simulink library "ODEHubs_components"  (R2020b)
settings: Solver=VariableStepAuto  StartTime=0.0  StopTime=10.0  RelTol=1e-3
values from neighbouring files (symbols this model uses):
  I = aux    [EH_definition_Simulink.m]
  O = aux    [EH_definition_Simulink.m]
undefined symbols (not defined in the file or in its folder): AbsorptionChiller, beta1, BiomassBoiler, Boiler, CN0, CombinedHeatAndPower, cpa, DesalinationPlant, dispatch_factor, DN0, efficiency, HeatPump, IrrigationPump, Low, Low1, Low2, Max_in, Max_out, Min_in, NanofiltrationPlant, PVModules, r_c, r_d, ReversibleHeatPump, SolarCollector, StorageSystem, T_muestreo, Tm, Up, Up1, Up2
(part 1 of 2)
settings Model: Creator=Usuario  LastModifiedBy=Javi
settings SFSimCC: CustomCodeUndefinedFunction=UseInterfaceOnly

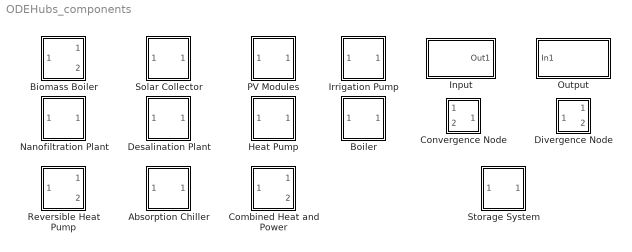
== system ODEHubs_components ==
  Absorption Chiller : Subsystem  mask{label=AbsorptionChiller, n=0, nI=1:1, tI="H", nO=1:1, tO="C", sO=1, Dimin=0, Dimax=0, Domin=0, Domax=0, nd=0}
      mask prompts: label "ID label:"; n "Number:"; Dimin "Input flow(s) lower bound (Dimin):"; Dimax "Input flow(s) upper bound (Dimax):"; Domin "Output flow(s) lower bounds (Domin):"; Domax "Output flow(s) upper bounds (Domax):"; nd "Conversion factor(s):"
      mask init:
      | %% Update user defined data from library
      | parent=libinfo(gcb);
      | if ~isempty(parent)
      | s_new=get_param(parent.ReferenceBlock,'UserData');
      | s_old=get_param(gcb,'UserData');
      | 
      | % Remove overlapping fields from first struct
      | s_merged = rmfield(s_old, intersect(fieldnames(s_old), fieldnames(s_new)));
      | 
      | % Obtain all unique names of remaining fields
      | names = [fieldnames(s_merged); fieldnames(s_new)];
      | 
      | % Merge both structs
      | s_merged = cell2struct([struct2cell(s_merged); struct2cell(s_new)], names, 1);
      | 
      | set_param(gcb,'UserData',s_merged);
      | set_param(gcb, 'UserDataPersistent', 'on');
      | end
      mask DialogControl DescGroupVar Prompt: Description
      mask DialogControl DescTextVar Prompt: Device description
      mask DialogControl Container3 Prompt: Device
      mask DialogControl ParameterGroupVar Prompt: Model
      mask Display:
      | %%Draw icon
      | ud = get_param(gcb,'UserData');
      | image(ud.icon);
      | 
      | 
      | %%Update label
      | subsys=find_system(gcs,...
      |     'LookUnderMasks','on',...
      |     'FollowLinks','on','BlockType','SubSystem');
      | UD=get_param(subsys,'UserData');
      | devs={};
      | for i=1:length(UD)
      |     if isfield(UD{i},'type')
      |         if UD{i}.type=='D'
      |             devs{end+1}=subsys{i}; %filter devices (D)
      |         end
      |     end
      | end
      | 
      | names=get_param(devs,'Name'); %all dev names
      | names=names(~cellfun(@isempty,erase(names,get_param(gcb,'Name')))); %remove this block
      | labels=matlab.lang.makeValidName(names); %all, but this block, dev labels
      | set_param(gcb,'label',matlab.lang.makeUniqueStrings(... %ensure uniqueness
      |                       matlab.lang.makeValidName(get_param(gcb,'Name')),...
      |                                                 labels))
  Biomass Boiler : Subsystem  mask{label=BiomassBoiler, n=0, nI=1:1, tI="B", nO=1:2, tO=["H";"G"], sO=[1 1], Dimin=0, Dimax=0, Domin=0, Domax=0, nd=0}
      mask prompts: label "ID label:"; n "Number:"; Dimin "Input flow(s) lower bound (Dimin):"; Dimax "Input flow(s) upper bound (Dimax):"; Domin "Output flow(s) lower bounds (Domin):"; Domax "Output flow(s) upper bounds (Domax):"; nd "Conversion factor(s):"
      mask init: same as ODEHubs_components/Absorption Chiller
      mask DialogControl DescGroupVar Prompt: Description
      mask DialogControl DescTextVar Prompt: Device description
      mask DialogControl Container3 Prompt: Device
      mask DialogControl ParameterGroupVar Prompt: Model
      mask Display:
      | %%Draw icon
      | ud = get_param(gcb,'UserData');
      | image(ud.icon);
      | 
      | 
      | %%Update label
      | subsys=find_system(gcs,...
      |     'LookUnderMasks','on',...
      |     'FollowLinks','on','BlockType','SubSystem');
      | UD=get_param(subsys,'UserData');
      | devs={};
      | for i=1:length(UD)
      |     if isfield(UD{i},'type')
      |         if UD{i}.type=='D'
      |             devs{end+1}=subsys{i}; %filter devices (D)
      |         end
      |     end
      | end
      | 
      | names=get_param(devs,'Name'); %all dev names
      | names=names(~cellfun(@isempty,erase(names,get_param(gcb,'Name')))); %remove this block
      | labels=matlab.lang.makeValidName(names); %all, but this block, dev labels
      | set_param(gcb,'label',matlab.lang.makeUniqueStrings(... %ensure uniqueness
      |                       matlab.lang.makeValidName(get_param(gcb,'Name')),...
      |                                                 labels))
  Boiler : Subsystem  mask{label=Boiler, n=0, nI=1:1, tI="P", nO=1:1, tO="H", sO=1, Dimin=0, Dimax=0, Domin=0, Domax=0, nd=0}
      mask prompts: label "ID label:"; n "Number:"; Dimin "Input flow(s) lower bound (Dimin):"; Dimax "Input flow(s) upper bound (Dimax):"; Domin "Output flow(s) lower bounds (Domin):"; Domax "Output flow(s) upper bounds (Domax):"; nd "Conversion factor(s):"
      mask init: same as ODEHubs_components/Absorption Chiller
      mask DialogControl DescGroupVar Prompt: Description
      mask DialogControl DescTextVar Prompt: Device description
      mask DialogControl Container3 Prompt: Device
      mask DialogControl ParameterGroupVar Prompt: Model
      mask Display:
      | %%Draw icon
      | ud = get_param(gcb,'UserData');
      | image(ud.icon);
      | 
      | 
      | %%Update label
      | subsys=find_system(gcs,...
      |     'LookUnderMasks','on',...
      |     'FollowLinks','on','BlockType','SubSystem');
      | UD=get_param(subsys,'UserData');
      | devs={};
      | for i=1:length(UD)
      |     if isfield(UD{i},'type')
      |         if UD{i}.type=='D'
      |             devs{end+1}=subsys{i}; %filter devices (D)
      |         end
      |     end
      | end
      | 
      | names=get_param(devs,'Name'); %all dev names
      | names=names(~cellfun(@isempty,erase(names,get_param(gcb,'Name')))); %remove this block
      | labels=matlab.lang.makeValidName(names); %all, but this block, dev labels
      | set_param(gcb,'label',matlab.lang.makeUniqueStrings(... %ensure uniqueness
      |                       matlab.lang.makeValidName(get_param(gcb,'Name')),...
      |                                                 labels))
  Combined Heat and Power : Subsystem  mask{label=CombinedHeatAndPower, n=0, nI=1:1, tI="P", nO=1:2, tO=["H";"E"], sO=[1 1], Dimin=0, Dimax=0, Domin=0, Domax=0, nd=0}
      mask prompts: label "ID label:"; n "Number:"; Dimin "Input flow(s) lower bound (Dimin):"; Dimax "Input flow(s) upper bound (Dimax):"; Domin "Output flow(s) lower bounds (Domin):"; Domax "Output flow(s) upper bounds (Domax):"; nd "Conversion factor(s):"
      mask init: same as ODEHubs_components/Absorption Chiller
      mask DialogControl DescGroupVar Prompt: Description
      mask DialogControl DescTextVar Prompt: Device description
      mask DialogControl Container3 Prompt: Device
      mask DialogControl ParameterGroupVar Prompt: Model
      mask Display:
      | %%Draw icon
      | ud = get_param(gcb,'UserData');
      | image(ud.icon);
      | 
      | 
      | %%Update label
      | subsys=find_system(gcs,...
      |     'LookUnderMasks','on',...
      |     'FollowLinks','on','BlockType','SubSystem');
      | UD=get_param(subsys,'UserData');
      | devs={};
      | for i=1:length(UD)
      |     if isfield(UD{i},'type')
      |         if UD{i}.type=='D'
      |             devs{end+1}=subsys{i}; %filter devices (D)
      |         end
      |     end
      | end
      | 
      | names=get_param(devs,'Name'); %all dev names
      | names=names(~cellfun(@isempty,erase(names,get_param(gcb,'Name')))); %remove this block
      | labels=matlab.lang.makeValidName(names); %all, but this block, dev labels
      | set_param(gcb,'label',matlab.lang.makeUniqueStrings(... %ensure uniqueness
      |                       matlab.lang.makeValidName(get_param(gcb,'Name')),...
      |                                                 labels))
  Convergence Node : Subsystem  mask{ID=CN0, n=0, Inputs=2}
      mask prompts: ID "ID label:"; n "Number:"; Inputs "Number of input flows:"
      mask init:
      | %% Update user defined data from library
      | parent=libinfo(gcb);
      | if ~isempty(parent)
      | s_new=get_param(parent.ReferenceBlock,'UserData');
      | s_old=get_param(gcb,'UserData');
      | 
      | % Remove overlapping fields from first struct
      | s_merged = rmfield(s_old, intersect(fieldnames(s_old), fieldnames(s_new)));
      | 
      | % Obtain all unique names of remaining fields
      | names = [fieldnames(s_merged); fieldnames(s_new)];
      | 
      | % Merge both structs
      | s_merged = cell2struct([struct2cell(s_merged); struct2cell(s_new)], names, 1);
      | 
      | set_param(gcb,'UserData',s_merged);
      | set_param(gcb, 'UserDataPersistent', 'on');
      | end
      | 
      | %%Update label
      | n = get_param(gcb,'n');
      | set_param(gcb,'ID',strcat('CN',num2str(n)));
      | 
      | %Update subsystem structure
      | blocks=find_system(gcb,...
      |         'LookUnderMasks','on',...
      |         'FollowLinks','on','BlockType','Inport');
      | lines=find_system(gcb,...
      |         'LookUnderMasks','on',...
      |         'FollowLinks','on','FindAll','On','type','line'); 
      | 
      | if Inputs~=length(blocks)
      |     
      |     %Delete all input ports
      |     delete_block(blocks)
      |     
      |     %Delete all the lines
      |     delete_line(lines)
      |     
      |     %Set sum block inputs
      |     set_param(strcat(gcb,'/Sum'),'Inputs',num2str(Inputs))
      |     
      |     %Build new inputs and lines
      |     for k=1:Inputs
      |         newblock=[gcb,char(strcat('/In',num2str(k)))];
      |         add_block('built-in/Inport',newblock);
      |         P0=get_param(newblock,'position');
      |         P=P0;
      |         P(1)=P0(1)+8; %left
      |         P(2)=P0(2)+18+k*20-100; %top
      |         P(3)=P0(3)-8; %right
      |         P(4)=P0(4)-18+k*20-100; %bottom
      |         set_param(newblock,'position',P);
      |         add_line(gcb,...
      |             strcat('In',num2str(k),'/1'),... %out
      |             strcat('Sum/',num2str(k)),...%in
      |             'autorouting','on')
      |     end
      |     add_line(gcb,...
      |         'Sum/1',... %out
      |         'Out1/1',...%in
      |         'autorouting','on')
      | end
      mask DialogControl DescGroupVar Prompt: Description
      mask DialogControl DescTextVar Prompt: Convergence node whose output is the sum of all the input flows
      mask Display:
      | icon=sprintf('\\fontname{Palatino Linotype}CN %s',n);
      | disp(icon, 'texmode','on');
      | plot(sin(0:0.0001:2*pi),cos(0:0.0001:2*pi))
  Desalination Plant : Subsystem  mask{label=DesalinationPlant, n=0, nI=1:1, tI="S", nO=1:1, tO="W", sO=1, Dimin=0, Dimax=0, Domin=0, Domax=0, nd=0}
      mask prompts: label "ID label:"; n "Number:"; Dimin "Input flow(s) lower bound (Dimin):"; Dimax "Input flow(s) upper bound (Dimax):"; Domin "Output flow(s) lower bounds (Domin):"; Domax "Output flow(s) upper bounds (Domax):"; nd "Conversion factor(s):"
      mask init: same as ODEHubs_components/Absorption Chiller
      mask DialogControl DescGroupVar Prompt: Description
      mask DialogControl DescTextVar Prompt: Device description
      mask DialogControl Container3 Prompt: Device
      mask DialogControl ParameterGroupVar Prompt: Model
      mask Display:
      | %%Draw icon
      | ud = get_param(gcb,'UserData');
      | image(ud.icon);
      | 
      | 
      | %%Update label
      | subsys=find_system(gcs,...
      |     'LookUnderMasks','on',...
      |     'FollowLinks','on','BlockType','SubSystem');
      | UD=get_param(subsys,'UserData');
      | devs={};
      | for i=1:length(UD)
      |     if isfield(UD{i},'type')
      |         if UD{i}.type=='D'
      |             devs{end+1}=subsys{i}; %filter devices (D)
      |         end
      |     end
      | end
      | 
      | names=get_param(devs,'Name'); %all dev names
      | names=names(~cellfun(@isempty,erase(names,get_param(gcb,'Name')))); %remove this block
      | labels=matlab.lang.makeValidName(names); %all, but this block, dev labels
      | set_param(gcb,'label',matlab.lang.makeUniqueStrings(... %ensure uniqueness
      |                       matlab.lang.makeValidName(get_param(gcb,'Name')),...
      |                                                 labels))
  Divergence Node : Subsystem  mask{ID=DN0, n=0, Outputs=2}
      mask prompts: ID "ID label:"; n "Number:"; Outputs "Number of output flows:"
      mask init:
      | %% Update user defined data from library
      | parent=libinfo(gcb);
      | if ~isempty(parent)
      | s_new=get_param(parent.ReferenceBlock,'UserData');
      | s_old=get_param(gcb,'UserData');
      | 
      | % Remove overlapping fields from first struct
      | s_merged = rmfield(s_old, intersect(fieldnames(s_old), fieldnames(s_new)));
      | 
      | % Obtain all unique names of remaining fields
      | names = [fieldnames(s_merged); fieldnames(s_new)];
      | 
      | % Merge both structs
      | s_merged = cell2struct([struct2cell(s_merged); struct2cell(s_new)], names, 1);
      | 
      | set_param(gcb,'UserData',s_merged);
      | set_param(gcb, 'UserDataPersistent', 'on');
      | end
      | 
      | %%Update label
      | n = get_param(gcb,'n');
      | set_param(gcb,'ID',strcat('DN',num2str(n)));
      | 
      | %%Update subsys structure
      | blocks1=find_system(gcb,...
      |         'LookUnderMasks','on',...
      |         'FollowLinks','on','BlockType','Gain');
      | blocks2=find_system(gcb,...
      |         'LookUnderMasks','on',...
      |         'FollowLinks','on','BlockType','Outport');
      | lines=find_system(gcb,...
      |         'LookUnderMasks','on',...
      |         'FollowLinks','on','FindAll','On','type','line'); 
      | 
      | if Outputs~=length(blocks2)
      |     
      |     %Delete all gain ports
      |     delete_block(blocks1)
      |     
      |     %Delete all output ports
      |     delete_block(blocks2)
      |     
      |     %Delete all the lines
      |     delete_line(lines)
      |     
      |     %Set mux and demux ports
      |     set_param(strcat(gcb,'/Mux'),'Inputs',num2str(Outputs))
      |     set_param(strcat(gcb,'/Demux'),'Outputs',num2str(Outputs))
      |     
      |     %Build new inputs and lines
      |     for k=1:Outputs
      |         
      |         %Add output ports
      |         newblock=[gcb,char(strcat('/Out',num2str(k)))];
      |         add_block('built-in/Outport',newblock);
      |         P0=get_param(newblock,'position');
      |         P=P0;
      |         P(1)=P0(1)+8; %left
      |         P(2)=P0(2)+18-80+k*20; %top
      |         P(3)=P0(3)-8; %right
      |         P(4)=P0(4)-18-80+k*20; %bottom
      |         set_param(newblock,'position',P);
      |         
      |         %Add gains
      |         newblock=[gcb,char(strcat('/Gain',num2str(k)))];
      |         add_block('built-in/Gain',newblock);
      |         P0=get_param(newblock,'position');
      |         P=P0;
      |         P(1)=P0(1)+8-40; %left
      |         P(2)=P0(2)+18-80+k*20; %top
      |         P(3)=P0(3)-8-40; %right
      |         P(4)=P0(4)-18-80+k*20; %bottom
      |         set_param(newblock,'position',P);
      |         %set equal default gains
      |         set_param(strcat(gcb,'/Gain',num2str(k)),'Gain',num2str(1/Outputs))
      |         
      |         %link in to mux ports
      |         add_line(gcb,...
      |             'In1/1',... %out
      |             strcat('Mux/',num2str(k)),...%in
      |             'autorouting','on')
      |         %link demux ports to gains
      |         add_line(gcb,...
      |             strcat('Demux/',num2str(k)),... %out
      |             strcat('Gain',num2str(k),'/1'),...%in
      |             'autorouting','on')
      |         %link gains to output ports
      |         add_line(gcb,...
      |             strcat('Gain',num2str(k),'/1'),... %out
      |             strcat('Out',num2str(k),'/1'),...%in
      |             'autorouting','on')
      |     end
      |     %link mux to demux
      |     add_line(gcb,...
      |         'Mux/1',... %in
      |         'Demux/1',...%out
      |         'autorouting','on')
      | end
      mask DialogControl DescGroupVar Prompt: Description
      mask DialogControl DescTextVar Prompt: Convergence node whose input is the sum of all the output flows
      mask Display:
      | icon=sprintf('\\fontname{Palatino Linotype}DN %s',n);
      | disp(icon, 'texmode','on');
      | plot(sin(0:0.0001:2*pi),cos(0:0.0001:2*pi))
  Heat Pump : Subsystem  mask{label=HeatPump, n=0, nI=1:1, tI="E", nO=1:1, tO="H", sO=1, Dimin=0, Dimax=0, Domin=0, Domax=0, nd=0}
      mask prompts: label "ID label:"; n "Number:"; Dimin "Input flow(s) lower bound (Dimin):"; Dimax "Input flow(s) upper bound (Dimax):"; Domin "Output flow(s) lower bounds (Domin):"; Domax "Output flow(s) upper bounds (Domax):"; nd "Conversion factor(s):"
      mask init: same as ODEHubs_components/Absorption Chiller
      mask DialogControl DescGroupVar Prompt: Description
      mask DialogControl DescTextVar Prompt: Device description
      mask DialogControl Container3 Prompt: Device
      mask DialogControl ParameterGroupVar Prompt: Model
      mask Display:
      | %%Draw icon
      | ud = get_param(gcb,'UserData');
      | image(ud.icon);
      | 
      | 
      | %%Update label
      | subsys=find_system(gcs,...
      |     'LookUnderMasks','on',...
      |     'FollowLinks','on','BlockType','SubSystem');
      | UD=get_param(subsys,'UserData');
      | devs={};
      | for i=1:length(UD)
      |     if isfield(UD{i},'type')
      |         if UD{i}.type=='D'
      |             devs{end+1}=subsys{i}; %filter devices (D)
      |         end
      |     end
      | end
      | 
      | names=get_param(devs,'Name'); %all dev names
      | names=names(~cellfun(@isempty,erase(names,get_param(gcb,'Name')))); %remove this block
      | labels=matlab.lang.makeValidName(names); %all, but this block, dev labels
      | set_param(gcb,'label',matlab.lang.makeUniqueStrings(... %ensure uniqueness
      |                       matlab.lang.makeValidName(get_param(gcb,'Name')),...
      |                                                 labels))
  Input : Subsystem  mask{label=I, n=0, t=I, l='', colour=[0  0  0], c=0, I_min=0, I_max=inf}
      mask prompts: label "ID label:"; n "Number:"; t "Define the type of resource:"; l "Label:"; c "Cost (c):"; I_min "Minimum input flow (Imin):"; I_max "Maximum input flow (Imax):"
      mask init:
      | %% Update user defined data from library
      | parent=libinfo(gcb);
      | if ~isempty(parent)
      | s_new=get_param(parent.ReferenceBlock,'UserData');
      | s_old=get_param(gcb,'UserData');
      | 
      | % Remove overlapping fields from first struct
      | s_merged = rmfield(s_old, intersect(fieldnames(s_old), fieldnames(s_new)));
      | 
      | % Obtain all unique names of remaining fields
      | names = [fieldnames(s_merged); fieldnames(s_new)];
      | 
      | % Merge both structs
      | s_merged = cell2struct([struct2cell(s_merged); struct2cell(s_new)], names, 1);
      | 
      | set_param(gcb,'UserData',s_merged);
      | set_param(gcb, 'UserDataPersistent', 'on');
      | end
      | 
      | %%Update label
      | t = get_param(gcb,'t');
      | l = get_param(gcb,'l');
      | l=l(2:end-1);
      | set_param(gcb,'label',sprintf('%s%s',t,l));
      mask TypeOptions t: A | B | C | D | E | F | G | H | I | J | K | L | M | N | O | P | Q | R | S | T | U | V | W | X | Y | Z
      mask DialogControl DescGroupVar Prompt: Description
      mask DialogControl DescTextVar Prompt: Input block of the energy hub
      mask DialogControl Container8 Prompt: Definition
      mask DialogControl col_gui Prompt: Set color for representation
      mask DialogControl col_gui Callback:
      | commandwindow;
      | col=uisetcolor([],'Color editor');
      | if length(col)~=3
      | else
      | col=['[',num2str(col),']'];
      | set_param(gcb,'colour',col);
      | end
      | open_system(gcb);
      mask DialogControl Container7 Prompt: Model
      mask Display:
      | t = get_param(gcb,'t');
      | l = get_param(gcb,'l');
      | l=l(2:end-1);
      | n = get_param(gcb,'n');
      | icon=sprintf('\\fontname{Palatino Linotype}%s%s (%s)',t,l,n);
      | disp(icon, 'texmode','on');
  Irrigation Pump : Subsystem  mask{label=IrrigationPump, n=0, nI=1:1, tI="W", nO=1:1, tO="W", sO=1, Dimin=0, Dimax=0, Domin=0, Domax=0, nd=0}
      mask prompts: label "ID label:"; n "Number:"; Dimin "Input flow(s) lower bound (Dimin):"; Dimax "Input flow(s) upper bound (Dimax):"; Domin "Output flow(s) lower bounds (Domin):"; Domax "Output flow(s) upper bounds (Domax):"; nd "Conversion factor(s):"
      mask init: same as ODEHubs_components/Absorption Chiller
      mask DialogControl DescGroupVar Prompt: Description
      mask DialogControl DescTextVar Prompt: Device description
      mask DialogControl Container3 Prompt: Device
      mask DialogControl ParameterGroupVar Prompt: Model
      mask Display:
      | %%Draw icon
      | ud = get_param(gcb,'UserData');
      | image(ud.icon);
      | 
      | 
      | %%Update label
      | subsys=find_system(gcs,...
      |     'LookUnderMasks','on',...
      |     'FollowLinks','on','BlockType','SubSystem');
      | UD=get_param(subsys,'UserData');
      | devs={};
      | for i=1:length(UD)
      |     if isfield(UD{i},'type')
      |         if UD{i}.type=='D'
      |             devs{end+1}=subsys{i}; %filter devices (D)
      |         end
      |     end
      | end
      | 
      | names=get_param(devs,'Name'); %all dev names
      | names=names(~cellfun(@isempty,erase(names,get_param(gcb,'Name')))); %remove this block
      | labels=matlab.lang.makeValidName(names); %all, but this block, dev labels
      | set_param(gcb,'label',matlab.lang.makeUniqueStrings(... %ensure uniqueness
      |                       matlab.lang.makeValidName(get_param(gcb,'Name')),...
      |                                                 labels))
  Nanofiltration Plant : Subsystem  mask{label=NanofiltrationPlant, n=0, nI=1:1, tI="D", nO=1:1, tO="W", sO=1, Dimin=0, Dimax=0, Domin=0, Domax=0, nd=0}
      mask prompts: label "ID label:"; n "Number:"; Dimin "Input flow(s) lower bound (Dimin):"; Dimax "Input flow(s) upper bound (Dimax):"; Domin "Output flow(s) lower bounds (Domin):"; Domax "Output flow(s) upper bounds (Domax):"; nd "Conversion factor(s):"
      mask init: same as ODEHubs_components/Absorption Chiller
      mask DialogControl DescGroupVar Prompt: Description
      mask DialogControl DescTextVar Prompt: Device description
      mask DialogControl Container3 Prompt: Device
      mask DialogControl ParameterGroupVar Prompt: Model
      mask Display:
      | %%Draw icon
      | ud = get_param(gcb,'UserData');
      | image(ud.icon);
      | 
      | 
      | %%Update label
      | subsys=find_system(gcs,...
      |     'LookUnderMasks','on',...
      |     'FollowLinks','on','BlockType','SubSystem');
      | UD=get_param(subsys,'UserData');
      | devs={};
      | for i=1:length(UD)
      |     if isfield(UD{i},'type')
      |         if UD{i}.type=='D'
      |             devs{end+1}=subsys{i}; %filter devices (D)
      |         end
      |     end
      | end
      | 
      | names=get_param(devs,'Name'); %all dev names
      | names=names(~cellfun(@isempty,erase(names,get_param(gcb,'Name')))); %remove this block
      | labels=matlab.lang.makeValidName(names); %all, but this block, dev labels
      | set_param(gcb,'label',matlab.lang.makeUniqueStrings(... %ensure uniqueness
      |                       matlab.lang.makeValidName(get_param(gcb,'Name')),...
      |                                                 labels))
  Output : Subsystem  mask{label=O, n=0, t=O, l='', colour=[0  0  0], dependance=none, prop=off, dev=0, devout=0, ms=off, f_label={"Power"}, st_label={"Energy"}, factor=1, lb=0, ub=0, st_factor=1, st_lb=0, st_ub=0, O=0, k=0, s=0, M_min=0, M_max=inf}
      mask prompts: label "ID label:"; n "Number:"; t "Define the type of resource:"; l "Label:"; dependance "Dependance on active flow:"; prop "Proportional demand"; dev "Select device or storage system:"; devout "Select device output:"; ms "Allow selling the resource attached to this output"; f_label "Flow label:"; st_label "Storage label:"; factor "Axis factor:"; lb "Lower limit:"; ub "Upper limit:"; st_factor "Axis factor:"; st_lb "Lower limit:"; st_ub "Upper limit:"; O "Output flow (O):"; k "Contant of proportionality (k):"; s "Price (s):"; M_min "Minimum sales flow (Mmin):"; M_max "Maximum sales flow (Mmax):"
      mask init: same as ODEHubs_components/Input
      mask TypeOptions t: A | B | C | D | E | F | G | H | I | J | K | L | M | N | O | P | Q | R | S | T | U | V | W | X | Y | Z
      mask TypeOptions dependance: none | device | charge | discharge
      mask Callback dependance:
      | d=get_param(gcb,'dependance');
      | p=Simulink.Mask.get(gcb);
      | 
      | if strcmp(d,'device')
      | %% Visulization
      | p.Parameters(strcmp(get_param(gcb,'MaskNames'),'dev')).set('Visible','on');
      | p.Parameters(strcmp(get_param(gcb,'MaskNames'),'devout')).set('Visible','on');
      | p.Parameters(strcmp(get_param(gcb,'MaskNames'),'prop')).set('Visible','on');
      | 
      | %%Update popout menu
      | p=Simulink.Mask.get(gcb);
      | subsys=find_system(gcs,...
      |     'LookUnderMasks','on',...
      |     'FollowLinks','on','BlockType','SubSystem');
      | UD=get_param(subsys,'UserData');
      | devs={};
      | for i=1:length(UD)
      |     if isfield(UD{i},'type')
      |         if UD{i}.type=='D'
      |             devs{end+1}=subsys{i}; %filter devices (D) or storage (S)
      |         end
      |     end
      | end
      | p.Parameters(strcmp(get_param(gcb,'MaskNames'),...
      |                     'dev')).TypeOptions=... %path to popout menu
      |                                         get_param(devs,'Name'); %dev names
      | 
      | elseif strcmp(d,'charge')
      | %% Visulization
      | p.Parameters(strcmp(get_param(gcb,'MaskNames'),'dev')).set('Visible','on');
      | p.Parameters(strcmp(get_param(gcb,'MaskNames'),'prop')).set('Visible','on');
      | p.Parameters(strcmp(get_param(gcb,'MaskNames'),'devout')).set('Visible','off');
      | set_param(gcb,'devout','0');
      | %%Update popout menu
      | p=Simulink.Mask.get(gcb);
      | subsys=find_system(gcs,...
      |     'LookUnderMasks','on',...
      |     'FollowLinks','on','BlockType','SubSystem');
      | UD=get_param(subsys,'UserData');
      | devs={};
      | %nns={};
      | for i=1:length(UD)
      |     if isfield(UD{i},'type')
      |         if UD{i}.type=='S'
      |             devs{end+1}=subsys{i}; %filter devices (D) or storage (S)
      |             %nns{end+1}=Simulink.Mask.get(subsys{i}).Parameters(1,2).Value; %obtains storage number
      |         end
      |     end
      | end
      | 
      | p.Parameters(strcmp(get_param(gcb,'MaskNames'),...
      |                     'dev')).TypeOptions=get_param(devs,'Name'); %dev names   %nns';... %path to popout menu
      | 
      | elseif strcmp(d,'discharge')
      | %% Visulization
      | p.Parameters(strcmp(get_param(gcb,'MaskNames'),'dev')).set('Visible','on');
      | p.Parameters(strcmp(get_param(gcb,'MaskNames'),'prop')).set('Visible','on');
      | p.Parameters(strcmp(get_param(gcb,'MaskNames'),'devout')).set('Visible','off');
      | set_param(gcb,'devout','0');
      | %%Update popout menu
      | p=Simulink.Mask.get(gcb);
      | subsys=find_system(gcs,...
      |     'LookUnderMasks','on',...
      |     'FollowLinks','on','BlockType','SubSystem');
      | UD=get_param(subsys,'UserData');
      | devs={};
      | %nns={};
      | for i=1:length(UD)
      |     if isfield(UD{i},'type')
      |         if UD{i}.type=='S'
      |             devs{end+1}=subsys{i}; %filter devices (D) or storage (S)
      |             %nns{end+1}=Simulink.Mask.get(subsys{i}).Parameters(1,2).Value; %obtains storage number
      |         end
      |     end
      | end
      | 
      | p.Parameters(strcmp(get_param(gcb,'MaskNames'),...
      |                     'dev')).TypeOptions=get_param(devs,'Name'); %dev names    %nns'; %path to popout menu
      | 
      | else
      | p.Parameters(strcmp(get_param(gcb,'MaskNames'),'dev')).set('Visible','off');
      | p.Parameters(strcmp(get_param(gcb,'MaskNames'),'devout')).set('Visible','off');
      | p.Parameters(strcmp(get_param(gcb,'MaskNames'),'prop')).set('Visible','off');
      | p.Parameters(strcmp(get_param(gcb,'MaskNames'),'k')).set('Visible','off');
      | 
      | %%Update popout menu
      | p=Simulink.Mask.get(gcb);
      | p.Parameters(strcmp(get_param(gcb,'MaskNames'),...
      |                     'dev')).TypeOptions=... %path to popout menu
      |                                         {'0'}; %dev names
      | 
      | set_param(gcb,'dev','0');
      | set_param(gcb,'devout','0');
      | set_param(gcb,'prop','off');
      | set_param(gcb,'k','0');
      | 
      | end
      mask Callback prop:
      | d=get_param(gcb,'dependance');
      | k=get_param(gcb,'prop');
      | p=Simulink.Mask.get(gcb);
      | 
      | if strcmp(d,'none')||strcmp(k,'off')
      | p.Parameters(strcmp(get_param(gcb,'MaskNames'),'O')).set('Visible','on');
      | p.Parameters(strcmp(get_param(gcb,'MaskNames'),'k')).set('Visible','off');
      | else
      | p.Parameters(strcmp(get_param(gcb,'MaskNames'),'O')).set('Visible','off');
      | p.Parameters(strcmp(get_param(gcb,'MaskNames'),'k')).set('Visible','on');
      | end
      mask TypeOptions dev: 0
      mask Callback dev:
      | %%Update popout menu
      | 
      | d=get_param(gcb,'dependance');
      | p=Simulink.Mask.get(gcb);
      | 
      | if strcmp(d,'device')
      | 
      |     %%Update popout menu
      |     p=Simulink.Mask.get(gcb);
      |     subsys=find_system(gcs,...
      |         'LookUnderMasks','on',...
      |         'FollowLinks','on','BlockType','SubSystem');
      |     UD=get_param(subsys,'UserData');
      |     devs={};
      |     for i=1:length(UD)
      |         if isfield(UD{i},'type')
      |             if UD{i}.type=='D'
      |                 devs{end+1}=subsys{i}; %filter devices (D) or storage (S)
      |             end
      |         end
      |     end
      |     p.Parameters(strcmp(get_param(gcb,'MaskNames'),...
      |         'dev')).TypeOptions=... %path to popout menu
      |         get_param(devs,'Name'); %dev names
      | 
      | elseif strcmp(d,'charge')
      | 
      |     set_param(gcb,'devout','0');
      | 
      |     %%Update popout menu
      |     p=Simulink.Mask.get(gcb);
      |     subsys=find_system(gcs,...
      |         'LookUnderMasks','on',...
      |         'FollowLinks','on','BlockType','SubSystem');
      |     UD=get_param(subsys,'UserData');
      |     devs={};
      |     for i=1:length(UD)
      |         if isfield(UD{i},'type')
      |             if UD{i}.type=='S'
      |                 devs{end+1}=subsys{i}; %filter devices (D) or storage (S)
      |             end
      |         end
      |     end
      | 
      |     p.Parameters(strcmp(get_param(gcb,'MaskNames'),...
      |         'dev')).TypeOptions=get_param(devs,'Name'); %dev names
      | 
      | elseif strcmp(d,'discharge')
      | 
      |     set_param(gcb,'devout','0');
      |     %%Update popout menu
      |     p=Simulink.Mask.get(gcb);
      |     subsys=find_system(gcs,...
      |         'LookUnderMasks','on',...
      |         'FollowLinks','on','BlockType','SubSystem');
      |     UD=get_param(subsys,'UserData');
      |     devs={};
      | 
      |     for i=1:length(UD)
      |         if isfield(UD{i},'type')
      |             if UD{i}.type=='S'
      |                 devs{end+1}=subsys{i}; %filter devices (D) or storage (S)
      |             end
      |         end
      |     end
      | 
      |     p.Parameters(strcmp(get_param(gcb,'MaskNames'),...
      |         'dev')).TypeOptions=get_param(devs,'Name'); %dev names
      | 
      | else
      |     % p.Parameters(strcmp(get_param(gcb,'MaskNames'),'dev')).set('Visible','off');
      |     % p.Parameters(strcmp(get_param(gcb,'MaskNames'),'devout')).set('Visible','off');
      |     % p.Parameters(strcmp(get_param(gcb,'MaskNames'),'prop')).set('Visible','off');
      |     % p.Parameters(strcmp(get_param(gcb,'MaskNames'),'k')).set('Visible','off');
      | 
      |     %%Update popout menu
      |     p=Simulink.Mask.get(gcb);
      |     p.Parameters(strcmp(get_param(gcb,'MaskNames'),...
      |         'dev')).TypeOptions=... %path to popout menu
      |         {'0'}; %dev names
      | 
      |     set_param(gcb,'dev','0');
      |     set_param(gcb,'devout','0');
      |     set_param(gcb,'prop','off');
      |     set_param(gcb,'k','0');
      | 
      | end
      mask TypeOptions devout: 0 | 1 | 2
      mask Callback ms:
      | ms=get_param(gcb,'ms');
      | p=Simulink.Mask.get(gcb);
      | if strcmp(ms,'on')
      |     %%Under-mask blocks
      |     replace_block(gcb,'Constant','FromWorkspace','noprompt');
      |     %%Model parameters visibility
      |     p.getDialogControl('ms_model').Visible='on';
      | else
      |     %%Under-mask blocks
      |     replace_block(gcb,'FromWorkspace','Constant','noprompt');
      |     c=find_system(gcb,...
      |         'LookUnderMasks','on',...
      |         'FollowLinks','on','BlockType','Constant');
      |     set_param(c{:},'Value','0');
      |     %%Model parameters visibility
      |     p.getDialogControl('ms_model').Visible='off';
      | end
      mask DialogControl DescGroupVar Prompt: Description
      mask DialogControl DescTextVar Prompt: Input block of the energy hub
      mask DialogControl Container11 Prompt: Definition
      mask DialogControl col_gui Prompt: Set color for representation
      mask DialogControl col_gui Callback:
      | commandwindow;
      | col=uisetcolor([],'Color editor');
      | if length(col)~=3
      | else
      | col=['[',num2str(col),']'];
      | set_param(gcb,'colour',col);
      | end
      | open_system(gcb);
      mask DialogControl Container12 Prompt: Representation
      mask DialogControl Container8_copy Prompt: Left axis
      mask DialogControl Container8 Prompt: Right axis
      mask DialogControl o_model Prompt: Model (output)
      mask DialogControl ms_model Prompt: Model (market sales)
      mask Display:
      | t = get_param(gcb,'t');
      | l = get_param(gcb,'l');
      | l=l(2:end-1);
      | n = get_param(gcb,'n');
      | icon=sprintf('\\fontname{Palatino Linotype}%s%s (%s)',t,l,n);
      | disp(icon, 'texmode','on');
  PV Modules : Subsystem  mask{label=PVModules, n=0, nI=1:1, tI="R", nO=1:1, tO="E", sO=1, Dimin=0, Dimax=0, Domin=0, Domax=0, nd=0}
      mask prompts: label "ID label:"; n "Number:"; Dimin "Input flow(s) lower bound (Dimin):"; Dimax "Input flow(s) upper bound (Dimax):"; Domin "Output flow(s) lower bounds (Domin):"; Domax "Output flow(s) upper bounds (Domax):"; nd "Conversion factor(s):"
      mask init: same as ODEHubs_components/Absorption Chiller
      mask DialogControl DescGroupVar Prompt: Description
      mask DialogControl DescTextVar Prompt: Device description
      mask DialogControl Container3 Prompt: Device
      mask DialogControl ParameterGroupVar Prompt: Model
      mask Display:
      | %%Draw icon
      | ud = get_param(gcb,'UserData');
      | image(ud.icon);
      | 
      | 
      | %%Update label
      | subsys=find_system(gcs,...
      |     'LookUnderMasks','on',...
      |     'FollowLinks','on','BlockType','SubSystem');
      | UD=get_param(subsys,'UserData');
      | devs={};
      | for i=1:length(UD)
      |     if isfield(UD{i},'type')
      |         if UD{i}.type=='D'
      |             devs{end+1}=subsys{i}; %filter devices (D)
      |         end
      |     end
      | end
      | 
      | names=get_param(devs,'Name'); %all dev names
      | names=names(~cellfun(@isempty,erase(names,get_param(gcb,'Name')))); %remove this block
      | labels=matlab.lang.makeValidName(names); %all, but this block, dev labels
      | set_param(gcb,'label',matlab.lang.makeUniqueStrings(... %ensure uniqueness
      |                       matlab.lang.makeValidName(get_param(gcb,'Name')),...
      |                                                 labels))
  Reversible Heat Pump : Subsystem  mask{label=ReversibleHeatPump, n=0, nI=1:1, tI="E", nO=1:2, tO=["C";"H"], sO=[1 2], Dimin=0, Dimax=0, Domin=0, Domax=0, nd=0}
      mask prompts: label "ID label:"; n "Number:"; Dimin "Input flow(s) lower bound (Dimin):"; Dimax "Input flow(s) upper bound (Dimax):"; Domin "Output flow(s) lower bounds (Domin):"; Domax "Output flow(s) upper bounds (Domax):"; nd "Conversion factor(s):"
      mask init: same as ODEHubs_components/Absorption Chiller
      mask DialogControl DescGroupVar Prompt: Description
      mask DialogControl DescTextVar Prompt: Device description
      mask DialogControl Container3 Prompt: Device
      mask DialogControl ParameterGroupVar Prompt: Model
      mask Display:
      | %%Draw icon
      | ud = get_param(gcb,'UserData');
      | image(ud.icon);
      | 
      | 
      | %%Update label
      | subsys=find_system(gcs,...
      |     'LookUnderMasks','on',...
      |     'FollowLinks','on','BlockType','SubSystem');
      | UD=get_param(subsys,'UserData');
      | devs={};
      | for i=1:length(UD)
      |     if isfield(UD{i},'type')
      |         if UD{i}.type=='D'
      |             devs{end+1}=subsys{i}; %filter devices (D)
      |         end
      |     end
      | end
      | 
      | names=get_param(devs,'Name'); %all dev names
      | names=names(~cellfun(@isempty,erase(names,get_param(gcb,'Name')))); %remove this block
      | labels=matlab.lang.makeValidName(names); %all, but this block, dev labels
      | set_param(gcb,'label',matlab.lang.makeUniqueStrings(... %ensure uniqueness
      |                       matlab.lang.makeValidName(get_param(gcb,'Name')),...
      |                                                 labels))
  Solar Collector : Subsystem  mask{label=SolarCollector, n=0, nI=1:1, tI="R", nO=1:1, tO="H", sO=1, Dimin=0, Dimax=0, Domin=0, Domax=0, nd=0}
      mask prompts: label "ID label:"; n "Number:"; Dimin "Input flow(s) lower bound (Dimin):"; Dimax "Input flow(s) upper bound (Dimax):"; Domin "Output flow(s) lower bounds (Domin):"; Domax "Output flow(s) upper bounds (Domax):"; nd "Conversion factor(s):"
      mask init: same as ODEHubs_components/Absorption Chiller
      mask DialogControl DescGroupVar Prompt: Description
      mask DialogControl DescTextVar Prompt: Device description
      mask DialogControl Container3 Prompt: Device
      mask DialogControl ParameterGroupVar Prompt: Model
      mask Display:
      | %%Draw icon
      | ud = get_param(gcb,'UserData');
      | image(ud.icon);
      | 
      | 
      | %%Update label
      | subsys=find_system(gcs,...
      |     'LookUnderMasks','on',...
      |     'FollowLinks','on','BlockType','SubSystem');
      | UD=get_param(subsys,'UserData');
      | devs={};
      | for i=1:length(UD)
      |     if isfield(UD{i},'type')
      |         if UD{i}.type=='D'
      |             devs{end+1}=subsys{i}; %filter devices (D)
      |         end
      |     end
      | end
      | 
      | names=get_param(devs,'Name'); %all dev names
      | names=names(~cellfun(@isempty,erase(names,get_param(gcb,'Name')))); %remove this block
      | labels=matlab.lang.makeValidName(names); %all, but this block, dev labels
      | set_param(gcb,'label',matlab.lang.makeUniqueStrings(... %ensure uniqueness
      |                       matlab.lang.makeValidName(get_param(gcb,'Name')),...
      |                                                 labels))
  Storage System : Subsystem  mask{label=StorageSystem, n=0, Qchmin=0, Qchmax=0, nch=0, Qdismin=0, Qdismax=0, ndis=0, Smin=0, Smax=0, ns=0, S0=0}
      mask prompts: label "ID label:"; n "Number:"; Qchmin "Charge flow lower bound (Qchmin):"; Qchmax "Charge flow upper bound (Qchmax):"; nch "Charge conversion factor (nch):"; Qdismin "Discharge flow lower bound (Qdismin):"; Qdismax "Discharge flow upper bound (Qdismax):"; ndis "Charge conversion factor (ndis):"; Smin "Capacity lower bound (Smin):"; Smax "Capacity upper bound (Smax):"; ns "Degradation conversion factor (ns):"; S0 "Storage initial state (S0):"
      mask init:
      | %% Update user defined data from library
      | parent=libinfo(gcb);
      | if ~isempty(parent)
      | s_new=get_param(parent.ReferenceBlock,'UserData');
      | s_old=get_param(gcb,'UserData');
      | 
      | % Remove overlapping fields from first struct
      | s_merged = rmfield(s_old, intersect(fieldnames(s_old), fieldnames(s_new)));
      | 
      | % Obtain all unique names of remaining fields
      | names = [fieldnames(s_merged); fieldnames(s_new)];
      | 
      | % Merge both structs
      | s_merged = cell2struct([struct2cell(s_merged); struct2cell(s_new)], names, 1);
      | 
      | set_param(gcb,'UserData',s_merged);
      | set_param(gcb, 'UserDataPersistent', 'on');
      | end
      | 
      | 
      | %% Update label
      | %get port handles
      | ph=get_param(gcb,'PortHandles');
      | %get the signal line associated with the output port of the inport
      | line = get_param(ph.Outport,'Line');
      | if line==-1 %Not conected to any block
      |     subsys=find_system(gcs,...
      |         'LookUnderMasks','on',...
      |         'FollowLinks','on','BlockType','SubSystem');
      |     UD=get_param(subsys,'UserData');
      |     devs={};
      |     for i=1:length(UD)
      |         if isfield(UD{i},'type')
      |             if UD{i}.type=='S'
      |                 devs{end+1}=subsys{i}; %filter storage devices (S)
      |             end
      |         end
      |     end
      |     
      |     names=get_param(devs,'Name'); %all dev names
      |     names=names(~cellfun(@isempty,erase(names,get_param(gcb,'Name')))); %remove this block
      |     labels=matlab.lang.makeValidName(names); %all, but this block, dev labels
      |     set_param(gcb,'label',matlab.lang.makeUniqueStrings(... %ensure uniqueness
      |         matlab.lang.makeValidName(get_param(gcb,'Name')),...
      |         labels))
      | 
      | else %Conected to any block
      |     %get the destination port handles for the signal
      |     dstport = get_param(line, 'Dstporthandle');
      |     %get the properties from the handle
      |     port = get(dstport);
      |     %get the block type
      |     UD=get_param(port.Parent,'UserData');
      |     if isfield(UD,'type')
      |         if UD.type=='O'
      |             set_param(gcb,'label',matlab.lang.makeValidName(get_param(gcb,'Name')))       
      |             set_param(gcb,'n',get_param(port.Parent,'n')) 
      |         else
      |             error('The storage system is not conected to any valid Output')
      |         end
      |     else
      |         error('The storage system is not conected to any valid Output')
      |     end
      |     
      | end
      mask DialogControl DescGroupVar Prompt: Description
      mask DialogControl DescTextVar Prompt: Device description
      mask DialogControl Container3 Prompt: Device
      mask DialogControl ParameterGroupVar Prompt: Model
      mask DialogControl Container6 Prompt: Charge
      mask DialogControl Container6_copy Prompt: Discharge
      mask DialogControl Container6_copy_copy Prompt: Storage
      mask Display:
      | %%Draw icon
      | ud = get_param(gcb,'UserData');
      | image(ud.icon);
      | 
      | %get port handles
      | ph=get_param(gcb,'PortHandles');
      | %get the signal line associated with the output port of the inport
      | line = get_param(ph.Outport,'Line');
      | 
      | if line==-1 %Not conected to any block
      |     set_param(gcb,'label',matlab.lang.makeValidName(get_param(gcb,'Name'))) %Rename var 'lavel'. Using the command
      |                                                                             %matlab.lang.makeUniqueStrings is unnecesary
      |                                                                             %because when the simulation starts, there are
      |                                                                             %funtions that fix it.
      |     set_param(gcb,'n','0')
      | 
      | else %Conected to any block
      |     %get the destination port handles for the signal
      |     dstport = get_param(line, 'Dstporthandle');
      |     %get the properties from the handle
      |     port = get(dstport);
      |     %get the block type
      |     UD=get_param(port.Parent,'UserData');
      | 
      |     if isfield(UD,'type')
      |         if UD.type=='O'
      |             set_param(gcb,'label',matlab.lang.makeValidName(get_param(gcb,'Name')))
      |             set_param(gcb,'n',get_param(port.Parent,'n'))
      | 
      |         else
      |              error('The storage system is not conected to any valid Output')
      |         end
      |     else
      |         error('The storage system is not conected to any valid Output')
      |     end
      | end

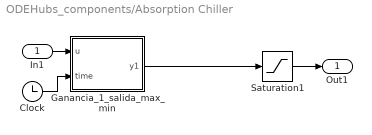
== system ODEHubs_components/Absorption Chiller ==
  In1 : Inport
  Clock : Clock
  Ganancia_1_salida_max_min : MATLAB Function  TreatAsAtomicUnit=on  mask{efficiency=efficiency, dispatch_factor=1, T_muestreo=T_muestreo, Min_in=Min_in, Max_in=Max_in}
      mask prompts: efficiency "Eficiencia"; dispatch_factor "Coeficiente de reparto"; T_muestreo "Tiempo de muestreo"; Min_in "Minimo de entrada"; Max_in "Minimo de salida"
  Saturation1 : Saturate  UpperLimit=Max_out  LowerLimit=-inf
  Out1 : Outport  VectorParamsAs1DForOutWhenUnconnected=off
  wires:
  In1/1 -> Ganancia_1_salida_max_min/1(u)
  Clock/1 -> Ganancia_1_salida_max_min/2(time)
  Ganancia_1_salida_max_min/1(y1) -> Saturation1/1
  Saturation1/1 -> Out1/1

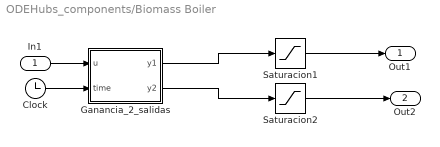
== system ODEHubs_components/Biomass Boiler ==
  In1 : Inport
  Clock : Clock
  Ganancia_2_salidas : MATLAB Function  TreatAsAtomicUnit=on  mask{efficiency=efficiency, T_muestreo=Tm, Max_in=Max_in, Min_in=Min_in, dispatch_factor=dispatch_factor}
      mask prompts: efficiency "Eficiencia"; T_muestreo "Tiempo de muestreo"; Max_in "Entrada máxima"; Min_in "Entrada mínima"; dispatch_factor "Coeficiente de reparto"
  Saturacion1 : Saturate  UpperLimit=Max_out(1)  LowerLimit=-inf
  Saturacion2 : Saturate  UpperLimit=Max_out(2)  LowerLimit=-inf
  Out1 : Outport  VectorParamsAs1DForOutWhenUnconnected=off
  Out2 : Outport  Port=2  VectorParamsAs1DForOutWhenUnconnected=off
  wires:
  Ganancia_2_salidas/2(y2) -> Saturacion2/1
  Ganancia_2_salidas/1(y1) -> Saturacion1/1
  Clock/1 -> Ganancia_2_salidas/2(time)
  In1/1 -> Ganancia_2_salidas/1(u)
  Saturacion2/1 -> Out2/1
  Saturacion1/1 -> Out1/1

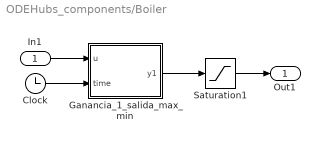
== system ODEHubs_components/Boiler ==
  In1 : Inport
  Clock : Clock
  Ganancia_1_salida_max_min : MATLAB Function  TreatAsAtomicUnit=on  mask{efficiency=0, dispatch_factor=1, T_muestreo=T_muestreo, Min_in=0, Max_in=0}
      mask prompts: efficiency "Eficiencia"; dispatch_factor "Coeficiente de reparto"; T_muestreo "Tiempo de muestreo"; Min_in "Minimo de entrada"; Max_in "Minimo de salida"
  Saturation1 : Saturate  UpperLimit=Max_out  LowerLimit=-inf
  Out1 : Outport  VectorParamsAs1DForOutWhenUnconnected=off
  wires:
  Saturation1/1 -> Out1/1
  Ganancia_1_salida_max_min/1(y1) -> Saturation1/1
  Clock/1 -> Ganancia_1_salida_max_min/2(time)
  In1/1 -> Ganancia_1_salida_max_min/1(u)

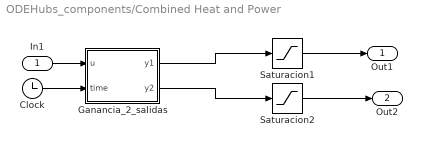
== system ODEHubs_components/Combined Heat and Power ==
  In1 : Inport
  Clock : Clock
  Ganancia_2_salidas : MATLAB Function  TreatAsAtomicUnit=on  mask{efficiency=[10 10], T_muestreo=T_muestreo, Max_in=1, Min_in=0, dispatch_factor=1}
      mask prompts: efficiency "Eficiencia"; T_muestreo "Tiempo de muestreo"; Max_in "Entrada máxima"; Min_in "Entrada mínima"; dispatch_factor "Coeficiente de reparto"
  Saturacion1 : Saturate  UpperLimit=Max_out(1)  LowerLimit=-inf
  Saturacion2 : Saturate  UpperLimit=Max_out(2)  LowerLimit=-inf
  Out1 : Outport  VectorParamsAs1DForOutWhenUnconnected=off
  Out2 : Outport  Port=2  VectorParamsAs1DForOutWhenUnconnected=off
  wires:
  Saturacion1/1 -> Out1/1
  Saturacion2/1 -> Out2/1
  In1/1 -> Ganancia_2_salidas/1(u)
  Clock/1 -> Ganancia_2_salidas/2(time)
  Ganancia_2_salidas/1(y1) -> Saturacion1/1
  Ganancia_2_salidas/2(y2) -> Saturacion2/1

== system ODEHubs_components/Convergence Node ==
  In1 : Inport
  In2 : Inport  Port=2
  Sum : Sum  Inputs=2
  Out1 : Outport
  wires:
  In1/1 -> Sum/1
  In2/1 -> Sum/2
  Sum/1 -> Out1/1

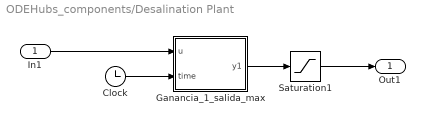
== system ODEHubs_components/Desalination Plant ==
  In1 : Inport
  Clock : Clock
  Ganancia_1_salida_max : MATLAB Function  TreatAsAtomicUnit=on  mask{Max_in=150, efficiency=1, T_muestreo=T_muestreo, dispatch_factor=beta1}
      mask prompts: Max_in "Máximo"; efficiency "Eficiencia"; T_muestreo "Tiempo de muestreo"; dispatch_factor "Coeficiente de reparto"
  Saturation1 : Saturate  UpperLimit=Max_out(1)  LowerLimit=-inf
  Out1 : Outport  VectorParamsAs1DForOutWhenUnconnected=off
  wires:
  In1/1 -> Ganancia_1_salida_max/1(u)
  Clock/1 -> Ganancia_1_salida_max/2(time)
  Ganancia_1_salida_max/1(y1) -> Saturation1/1
  Saturation1/1 -> Out1/1
